simulink model "Model_pH_and_level_V1"  (Simulink 8.3)
settings: Solver=ode1  SolverMode=SingleTasking  StartTime=0.0  StopTime=Tsim  FixedStep=delta_sim  RelTol=1e-7
values from neighbouring files (symbols this model uses):
  b = 0    [Configuring_pH_and_level_model.m]
  delta_sim = 0.05    [Simulating_pH_and_level_model.m]
  e1 = 50    [Configuring_pH_and_level_model.m]
  e2 = 300    [Configuring_pH_and_level_model.m]
  filter_estimator1 = 1    [Configuring_pH_and_level_model.m]
  filter_estimator2 = 1    [Configuring_pH_and_level_model.m]
  filter_estimator3 = 1    [Configuring_pH_and_level_model.m]
  filter_estimator4 = 1    [Configuring_pH_and_level_model.m]
  filter_estimator5 = 1    [Configuring_pH_and_level_model.m]
  filter_estimator6 = 1    [Configuring_pH_and_level_model.m]
  filtro_Kp = fir1(5,1/50)    [Configuring_pH_and_level_model.m]
  filtro_med_F_TAPI = 1    [Configuring_pH_and_level_model.m]
  filtro_med_F_TASI = 1    [Configuring_pH_and_level_model.m]
  filtro_med_pH = 1    [Configuring_pH_and_level_model.m]
  filtro_Ti = fir1(5,1/50)    [Configuring_pH_and_level_model.m]
  h_max_TR_m = 0.5    [Configuring_pH_and_level_model.m]
  h_nom = 75    [Configuring_pH_and_level_model.m]
  I_l = 271.52    [Configuring_pH_and_level_model.m]
  K_meter_flow = 3600    [Configuring_pH_and_level_model.m]
  K_meter_level = 1    [Configuring_pH_and_level_model.m]
  K_meter_pH = 1    [Configuring_pH_and_level_model.m]
  Kc = 3.5    [Configuring_pH_and_level_model.m]
  Kn = 100/14    (= 7.14285714286)    [Configuring_pH_and_level_model.m]
  Kv = 11e-2    (= 0.11)    [Configuring_pH_and_level_model.m]
  mv0 = 50    [Configuring_pH_and_level_model.m]
  N = 1/500    (= 0.002)    [Configuring_pH_and_level_model.m]
  P_l = 11.65    [Configuring_pH_and_level_model.m]
  pH_nom = 7    [Configuring_pH_and_level_model.m]
  pka1_CH3COOH = interp1(Temp,pK_CH3COOH,T)    [Configuring_pH_and_level_model.m]
  pka1_H2CO3 = interp1(Temp,pK_H2CO3,T)    [Configuring_pH_and_level_model.m]
  pka1_H3PO4 = interp1(Temp,pK_H3PO4,T)    [Configuring_pH_and_level_model.m]
  pka1_NH4 = interp1(Temp,pK_NH4,T)    [Configuring_pH_and_level_model.m]
  pka2_H2CO3 = interp1(Temp,pK_HCO3,T)    [Configuring_pH_and_level_model.m]
  pka2_H3PO4 = interp1(Temp,pK_H2PO4,T)    [Configuring_pH_and_level_model.m]
  pka3_H3PO4 = interp1(Temp,pK_HPO4,T)    [Configuring_pH_and_level_model.m]
  pKw = interp1(Temp,pK_H2O,T)    [Configuring_pH_and_level_model.m]
  Q_ap_nom = 49/3600    (= 0.0136111111111)    [Configuring_pH_and_level_model.m]
  Qb_nom = c_HCl/c_NaOH*Q_ap_nom    (= 0.00412773748633)    [Configuring_pH_and_level_model.m]
  seed_noise_level = 12345    [Configuring_pH_and_level_model.m]
  seed_noise_pH = 67890    [Configuring_pH_and_level_model.m]
  seed_noise_Q_ap = 357    [Configuring_pH_and_level_model.m]
  seed_noise_Q_as = 349    [Configuring_pH_and_level_model.m]
  T_noise_level = 2    [Configuring_pH_and_level_model.m]
  T_noise_pH = 3    [Configuring_pH_and_level_model.m]
  T_PWM = 10    [Configuring_pH_and_level_model.m]
  tau_meter_flow = 1.4    [Configuring_pH_and_level_model.m]
  tau_meter_level = 16    [Configuring_pH_and_level_model.m]
  tau_meter_pH = 5    [Configuring_pH_and_level_model.m]
  Td = 120    [Configuring_pH_and_level_model.m]
  td_meter_flow = 3.5    [Configuring_pH_and_level_model.m]
  td_meter_level = 6    [Configuring_pH_and_level_model.m]
  td_meter_pH = 3.5    [Configuring_pH_and_level_model.m]
  Ti = 150    [Configuring_pH_and_level_model.m]
  Tmix = 1.34    [Configuring_pH_and_level_model.m]
  Ts = 0.5    [Simulating_pH_and_level_model.m]
  Ts_F_TAPI = 1    [Configuring_pH_and_level_model.m]
  Ts_F_TASI = 1    [Configuring_pH_and_level_model.m]
  Ts_Kp = 5    [Configuring_pH_and_level_model.m]
  Ts_pH_m = 1    [Configuring_pH_and_level_model.m]
  Ts_Ti = 5    [Configuring_pH_and_level_model.m]
  Ts_w1 = 1    [Configuring_pH_and_level_model.m]
  Ts_w2 = 1    [Configuring_pH_and_level_model.m]
  Ts_w3 = 1    [Configuring_pH_and_level_model.m]
  Ts_w4 = 1    [Configuring_pH_and_level_model.m]
  Ts_w5 = 1    [Configuring_pH_and_level_model.m]
  Ts_w6 = 25    [Configuring_pH_and_level_model.m]
  V0_CSTR = V_max_CSTR*h_nom/h_max_TR    (= 46.3491936722)    [Configuring_pH_and_level_model.m]
  V_max_CSTR = A_util_TR*h_max_TR_m*1000    (= 61.7989248962)    [Configuring_pH_and_level_model.m]
  var_noise_level = 1.1e-3    (= 0.0011)    [Configuring_pH_and_level_model.m]
  var_noise_pH = 6.25e-5    (= 6.25e-05)    [Configuring_pH_and_level_model.m]
  var_noise_Q_ap = 1.56e-2    (= 0.0156)    [Configuring_pH_and_level_model.m]
  var_noise_Q_as = 1.56e-2    (= 0.0156)    [Configuring_pH_and_level_model.m]
  Vm = 0.836    [Configuring_pH_and_level_model.m]
  w1_ff_tap = 0.0056    [Configuring_pH_and_level_model.m]
  w1_ff_tas = 0    [Configuring_pH_and_level_model.m]
  w1_ff_tbb = -0.0185    [Configuring_pH_and_level_model.m]
  w2_ff_tap = 0.5e-4    (= 5e-05)    [Configuring_pH_and_level_model.m]
  w2_ff_tbb = 0.5e-4    (= 5e-05)    [Configuring_pH_and_level_model.m]
  w3_ff_tap = 3e-4    (= 0.0003)    [Configuring_pH_and_level_model.m]
  w3_ff_tas = 3e-4    (= 0.0003)    [Configuring_pH_and_level_model.m]
  w3_ff_tbb = 3e-4    (= 0.0003)    [Configuring_pH_and_level_model.m]
  w4_ff_tap = 2e-4    (= 0.0002)    [Configuring_pH_and_level_model.m]
  w4_ff_tas = 2e-4    (= 0.0002)    [Configuring_pH_and_level_model.m]
  w4_ff_tbb = 2e-4    (= 0.0002)    [Configuring_pH_and_level_model.m]
  w_ap1 = c_HCl    (= 0.0055861204494)    [Configuring_pH_and_level_model.m]
  w_ap2 = c_CH3COOH_r    (= 0.0001)    [Configuring_pH_and_level_model.m]
  w_ap3 = c_H2CO3_r    (= 0.0009)    [Configuring_pH_and_level_model.m]
  w_ap4 = c_NH4    (= 0.0002)    [Configuring_pH_and_level_model.m]
  w_ap5 = c_H3PO4    (= 1e-05)    [Configuring_pH_and_level_model.m]
  w_as1 = 0    [Configuring_pH_and_level_model.m]
  w_as2 = c_CH3COOH    (= 0.00676612574825)    [Configuring_pH_and_level_model.m]
  w_as3 = c_H2CO3_r    (= 0.0009)    [Configuring_pH_and_level_model.m]
  w_as4 = c_NH4    (= 0.0002)    [Configuring_pH_and_level_model.m]
  w_as5 = c_H3PO4    (= 1e-05)    [Configuring_pH_and_level_model.m]
  w_b1 = -c_NaOH    (= -0.0184200924523)    [Configuring_pH_and_level_model.m]
  w_b2 = c_CH3COOH_r    (= 0.0001)    [Configuring_pH_and_level_model.m]
  w_b3 = c_H2CO3    (= 0.0005)    [Configuring_pH_and_level_model.m]
  w_b4 = c_NH4    (= 0.0002)    [Configuring_pH_and_level_model.m]
  w_b5 = c_H3PO4    (= 1e-05)    [Configuring_pH_and_level_model.m]
  w_fb_tap = [w1_ff_tap w2_ff_tap w3_ff_tap w4_ff_tap]    [Configuring_pH_and_level_model.m]
  w_fb_tas = [w1_ff_tas 0 w3_ff_tas w4_ff_tas]    [Configuring_pH_and_level_model.m]
  w_r1_0 = [w1_r1_0; c_CH3COOH_r; c_H2CO3_r; c_NH4; c_H3PO4]    [Configuring_pH_and_level_model.m]
  x_MV_pump = [0 10 20 40 50 60 80 100]    [Configuring_pH_and_level_model.m]
  y_Q_pump = Q_l_h/3600    [Configuring_pH_and_level_model.m]
libraries: simulink x6, simulink_extras x4
(part 2 of 2)

== system Model_pH_and_level_V1/pH controller/controller/FB/Calculo Parâmetros Cont. ==
  note: F(1+T(pH))
  w : Inport
  pH_sp : Inport  Port=2
  F_TAPI : Inport  Port=3
  F_TASI : Inport  Port=4
  Constant1 : Constant  Value=1/e1
  Constant2 : Constant  Value=1/e2
  Constant3 : Constant  Value=46.35
  Constant4 : Constant  Value=e1
  Constant5 : Constant  Value=e2
  Constant6 : Constant
  Constant7 : Constant  Value=46.35
  Constant8 : Constant
  Divide1 : Product  Inputs=*/
  Divide4 : Product  Inputs=*/
  Gain2 : Gain  Gain=1/3600
  Gain3 : Gain  Gain=1/3600
  Product1 : Product
  Product2 : Product  Inputs=3
  Product4 : Product
  Sum{1..2,4,12} (4 alike) : Sum
  Sum3 : Sum  Inputs=+-
  Sum6 : Sum  Inputs=-+
  T(pH_sp) : Subsystem
  1/Ti : Outport
  Kp : Outport  Port=2
  wires:
  Sum12/1 -> Product4/2
  F_TAPI/1 -> Gain2/1
  F_TASI/1 -> Gain3/1
  Constant6/1 -> Sum1/2
  T(pH_sp)/1(T(pH_sp)) -> Sum1/1
  Constant4/1 -> Product2/2, Sum4/1
  Constant5/1 -> Product2/3, Sum4/2
  Product2/1 -> Divide4/1
  Constant2/1 -> Sum2/2
  Sum4/1 -> Sum6/2
  Sum2/1 -> Product1/1
  Constant3/1 -> Product1/2
  Gain2/1 -> Sum12/1, T(pH_sp)/3(F_TAPI)
  Sum1/1 -> Product4/1
  Constant1/1 -> Sum2/1
  Constant7/1 -> Divide4/2
  Product4/1 -> Sum3/2, Product2/1
  Sum3/1 -> Kp/1
  Divide4/1 -> Sum6/1
  Product1/1 -> Sum3/1
  Gain3/1 -> Sum12/2, T(pH_sp)/4(F_TASI)
  pH_sp/1 -> T(pH_sp)/2(pH_sp)
  w/1 -> T(pH_sp)/1(w)
  Divide1/1 -> 1/Ti/1
  Sum6/1 -> Divide1/2
  Constant8/1 -> Divide1/1

== system Model_pH_and_level_V1/pH controller/controller/FB/T(pH) ==
  w : Inport
  pH : Inport  Port=2
  pH_sp : Inport  Port=3
  F_TAPI : Inport  Port=4
  F_TASI : Inport  Port=5
  Constant1 : Constant
  Constant5 : Constant
  Gain2 : Gain  Gain=1/3600
  Gain3 : Gain  Gain=1/3600
  Sum1 : Sum
  Sum2 : Sum
  Sum5 : Sum  Inputs=+-
  T(pH) : Subsystem
  T(pH_sp) : Subsystem
  1+T(pH_sp) : Outport
  T(pH_sp)-T(pH) : Outport  Port=2
  1+T(pH) : Outport  Port=3
  wires:
  w/1 -> T(pH)/1(w), T(pH_sp)/1(w)
  pH_sp/1 -> T(pH_sp)/2(pH_sp)
  Gain3/1 -> T(pH)/4(F_TASI), T(pH_sp)/4(F_TASI)
  Gain2/1 -> T(pH_sp)/3(F_TAPI), T(pH)/3(F_TAPI)
  F_TASI/1 -> Gain3/1
  F_TAPI/1 -> Gain2/1
  pH/1 -> T(pH)/2(pH)
  T(pH_sp)/1(T(pH_sp)) -> Sum1/2, Sum5/1
  T(pH)/1(T(pH)) -> Sum2/1, Sum5/2
  Constant5/1 -> Sum1/1
  Constant1/1 -> Sum2/2
  Sum5/1 -> T(pH_sp)-T(pH)/1
  Sum1/1 -> 1+T(pH_sp)/1
  Sum2/1 -> 1+T(pH)/1

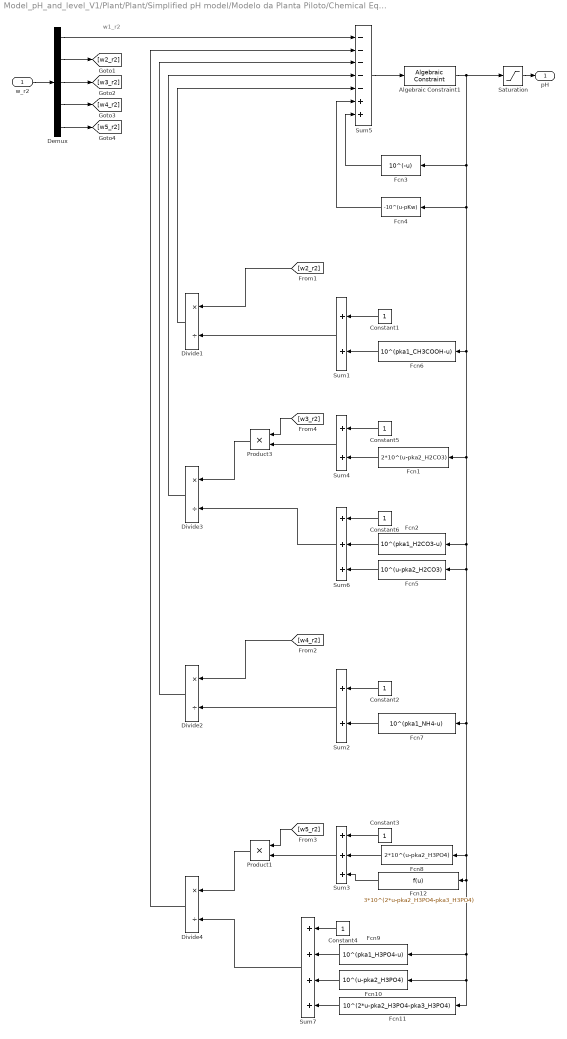
== system Model_pH_and_level_V1/Plant/Plant/Simplified pH model/Modelo da Planta Piloto/Chemical Equilibrium ==
  note: w1_r2
  w_r2 : Inport
  Algebraic Constraint1 : simulink/Math Operations/Algebraic Constraint  z0=7
  Constant{1..6} (6 alike) : Constant
  Demux : Demux  Outputs=5
  Divide{1..4} (4 alike) : Product  Inputs=*/
  Fcn1 : Fcn  Expr=2*10^(u-pka2_H2CO3)
  Fcn10 : Fcn  Expr=10^(u-pka2_H3PO4)
  Fcn11 : Fcn  Expr=10^(2*u-pka2_H3PO4-pka3_H3PO4)
  Fcn12 : Fcn  Expr=3*10^(2*u-pka2_H3PO4-pka3_H3PO4)
  Fcn2 : Fcn  Expr=10^(pka1_H2CO3-u)
  Fcn3 : Fcn  Expr=10^(-u)
  Fcn4 : Fcn  Expr=-10^(u-pKw)
  Fcn5 : Fcn  Expr=10^(u-pka2_H2CO3)
  Fcn6 : Fcn  Expr=10^(pka1_CH3COOH-u)
  Fcn7 : Fcn  Expr=10^(pka1_NH4-u)
  Fcn8 : Fcn  Expr=2*10^(u-pka2_H3PO4)
  Fcn9 : Fcn  Expr=10^(pka1_H3PO4-u)
  Product1 : Product
  Product3 : Product
  Saturation : Saturate  UpperLimit=14  LowerLimit=0
  Sum1 : Sum
  Sum2 : Sum
  Sum3 : Sum  Inputs=+++
  Sum4 : Sum
  Sum5 : Sum  Inputs=-----++
  Sum6 : Sum  Inputs=+++
  Sum7 : Sum  Inputs=++++
  pH : Outport
  wires:
  Sum4/1 -> Product3/2
  Product3/1 -> Divide3/1
  Constant5/1 -> Sum4/1
  Algebraic Constraint1/1 -> Fcn3/1, Fcn6/1, Fcn1/1, Fcn2/1, Fcn5/1, Fcn12/1, Fcn9/1, Fcn10/1, Fcn11/1, Fcn8/1, Fcn7/1, Fcn4/1, Saturation/1
  Fcn5/1 -> Sum6/3
  Sum6/1 -> Divide3/2
  Sum5/1 -> Algebraic Constraint1/1
  Fcn1/1 -> Sum4/2
  Fcn2/1 -> Sum6/2
  Constant6/1 -> Sum6/1
  Saturation/1 -> pH/1
  w_r2/1 -> Demux/1
  Demux/1 -> Sum5/1
  Demux/2 -> [w2_r2]
  Demux/3 -> [w3_r2]
  [w3_r2] -> Product3/1
  [w2_r2] -> Divide1/1
  Sum1/1 -> Divide1/2
  Fcn6/1 -> Sum1/2
  Constant1/1 -> Sum1/1
  Demux/4 -> [w4_r2]
  [w4_r2] -> Divide2/1
  Sum2/1 -> Divide2/2
  Fcn7/1 -> Sum2/2
  Constant2/1 -> Sum2/1
  Fcn3/1 -> Sum5/7
  Fcn4/1 -> Sum5/6
  Sum3/1 -> Product1/2
  Product1/1 -> Divide4/1
  Constant3/1 -> Sum3/1
  Fcn10/1 -> Sum7/3
  Sum7/1 -> Divide4/2
  Fcn8/1 -> Sum3/2
  Fcn9/1 -> Sum7/2
  Constant4/1 -> Sum7/1
  [w5_r2] -> Product1/1
  Fcn11/1 -> Sum7/4
  Demux/5 -> [w5_r2]
  Divide1/1 -> Sum5/5
  Divide3/1 -> Sum5/4
  Divide2/1 -> Sum5/3
  Divide4/1 -> Sum5/2
  Fcn12/1 -> Sum3/3

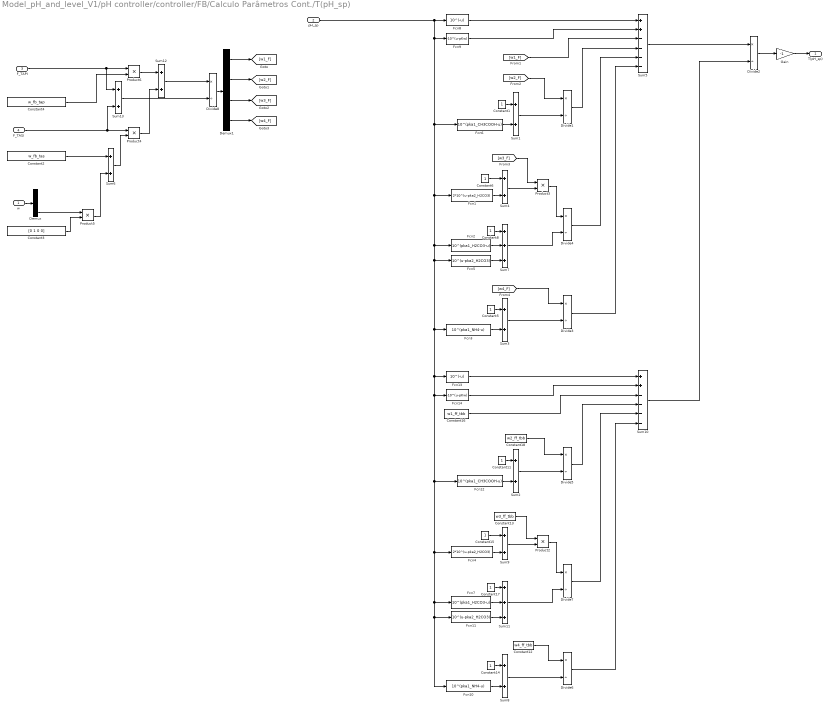
== system Model_pH_and_level_V1/pH controller/controller/FB/Calculo Parâmetros Cont./T(pH_sp) ==
  w : Inport
  pH_sp : Inport  Port=2
  F_TAPI : Inport  Port=3
  F_TASI : Inport  Port=4
  Constant{1,5..6,8,11,14..15,17} (8 alike) : Constant
  Constant12 : Constant  Value=w4_ff_tbb
  Constant13 : Constant  Value=w3_ff_tbb
  Constant16 : Constant  Value=w1_ff_tbb
  Constant18 : Constant  Value=w2_ff_tbb
  Constant2 : Constant  Value=w_fb_tas
  Constant3 : Constant  Value=[0 1 0 0]
  Constant4 : Constant  Value=w_fb_tap
  Demux : Demux  Outputs=6
  Demux1 : Demux
  Divide{1..8} (8 alike) : Product  Inputs=*/
  Fcn1 : Fcn  Expr=2*10^(u-pka2_H2CO3)
  Fcn10 : Fcn  Expr=10^(pka1_NH4-u)
  Fcn11 : Fcn  Expr=10^(u-pka2_H2CO3)
  Fcn12 : Fcn  Expr=10^(pka1_CH3COOH-u)
  Fcn13 : Fcn  Expr=10^(-u)
  Fcn14 : Fcn  Expr=-10^(u-pKw)
  Fcn2 : Fcn  Expr=10^(pka1_H2CO3-u)
  Fcn3 : Fcn  Expr=10^(pka1_NH4-u)
  Fcn4 : Fcn  Expr=2*10^(u-pka2_H2CO3)
  Fcn5 : Fcn  Expr=10^(u-pka2_H2CO3)
  Fcn6 : Fcn  Expr=10^(pka1_CH3COOH-u)
  Fcn7 : Fcn  Expr=10^(pka1_H2CO3-u)
  Fcn8 : Fcn  Expr=10^(-u)
  Fcn9 : Fcn  Expr=-10^(u-pKw)
  Gain : Gain  Gain=-1
  Product{2..4,6} (4 alike) : Product
  Product5 : Product  SampleTime=Ts_w5
  Sum{1..4,6,8..9,12..13} (9 alike) : Sum
  Sum10 : Sum  Inputs=++----
  Sum11 : Sum  Inputs=+++
  Sum5 : Sum  Inputs=++----
  Sum7 : Sum  Inputs=+++
  T(pH_sp) : Outport
  wires:
  Gain/1 -> T(pH_sp)/1
  w/1 -> Demux/1
  Constant18/1 -> Divide5/1
  Fcn7/1 -> Sum11/2
  Fcn4/1 -> Sum9/2
  Divide7/1 -> Sum10/5
  Sum10/1 -> Divide2/2
  Constant14/1 -> Sum8/1
  Constant12/1 -> Divide6/1
  Constant11/1 -> Sum2/1
  Fcn12/1 -> Sum2/2
  Sum2/1 -> Divide5/2
  Constant16/1 -> Sum10/3
  Divide6/1 -> Sum10/6
  Constant13/1 -> Product2/1
  Divide5/1 -> Sum10/4
  Constant17/1 -> Sum11/1
  Fcn13/1 -> Sum10/1
  Fcn10/1 -> Sum8/2
  Fcn14/1 -> Sum10/2
  Sum8/1 -> Divide6/2
  Fcn9/1 -> Sum5/2
  Fcn11/1 -> Sum11/3
  Sum11/1 -> Divide7/2
  Sum9/1 -> Product2/2
  pH_sp/1 -> Fcn8/1, Fcn9/1, Fcn6/1, Fcn1/1, Fcn2/1, Fcn3/1, Fcn10/1, Fcn11/1, Fcn7/1, Fcn4/1, Fcn12/1, Fcn14/1, Fcn13/1, Fcn5/1
  Divide4/1 -> Sum5/5
  Divide1/1 -> Sum5/4
  Sum5/1 -> Divide2/1
  Divide3/1 -> Sum5/6
  Constant15/1 -> Sum9/1
  [w4_F] -> Divide3/1
  Fcn3/1 -> Sum3/2
  [w2_F] -> Divide1/1
  Sum3/1 -> Divide3/2
  Product2/1 -> Divide7/1
  Fcn8/1 -> Sum5/1
  Constant5/1 -> Sum3/1
  Constant1/1 -> Sum1/1
  Sum4/1 -> Product3/2
  Fcn1/1 -> Sum4/2
  Fcn2/1 -> Sum7/2
  Sum1/1 -> Divide1/2
  Fcn6/1 -> Sum1/2
  Constant6/1 -> Sum4/1
  Sum7/1 -> Divide4/2
  Constant8/1 -> Sum7/1
  Fcn5/1 -> Sum7/3
  Product3/1 -> Divide4/1
  [w1_F] -> Sum5/3
  [w3_F] -> Product3/1
  F_TASI/1 -> Sum13/2, Product4/1
  Constant3/1 -> Product5/2
  Product5/1 -> Sum6/2
  Constant2/1 -> Sum6/1
  Sum6/1 -> Product4/2
  F_TAPI/1 -> Sum13/1, Product6/1
  Constant4/1 -> Product6/2
  Product6/1 -> Sum12/1
  Product4/1 -> Sum12/2
  Sum12/1 -> Divide8/1
  Sum13/1 -> Divide8/2
  Divide8/1 -> Demux1/1
  Demux1/1 -> [w1_F]
  Demux1/2 -> [w2_F]
  Demux1/3 -> [w3_F]
  Demux1/4 -> [w4_F]
  Divide2/1 -> Gain/1
  Demux/6 -> Product5/1

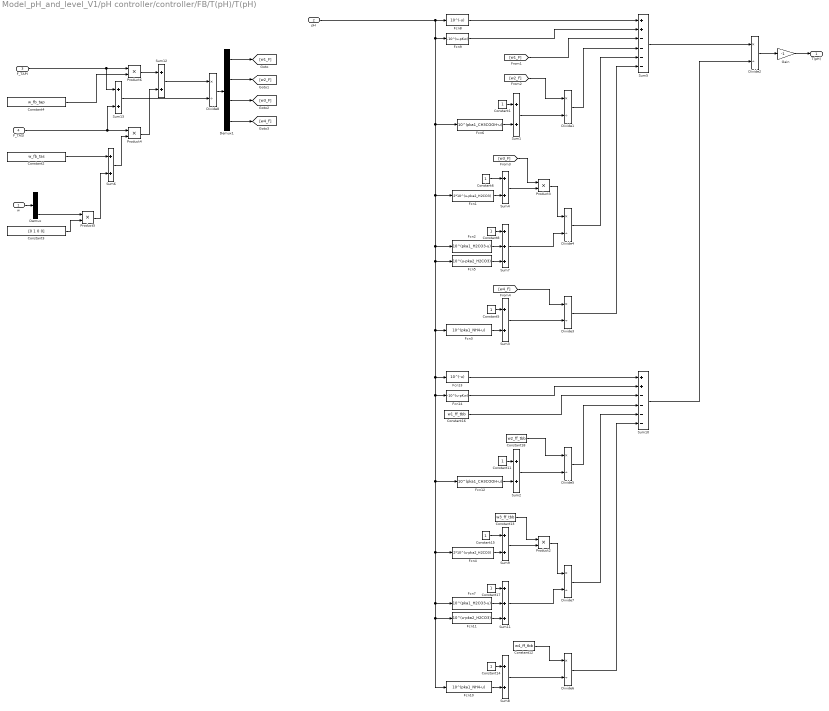
== system Model_pH_and_level_V1/pH controller/controller/FB/T(pH)/T(pH) ==
  w : Inport
  pH : Inport  Port=2
  F_TAPI : Inport  Port=3
  F_TASI : Inport  Port=4
  Constant{1,5..6,8,11,14..15,17} (8 alike) : Constant
  Constant12 : Constant  Value=w4_ff_tbb
  Constant13 : Constant  Value=w3_ff_tbb
  Constant16 : Constant  Value=w1_ff_tbb
  Constant18 : Constant  Value=w2_ff_tbb
  Constant2 : Constant  Value=w_fb_tas
  Constant3 : Constant  Value=[0 1 0 0]
  Constant4 : Constant  Value=w_fb_tap
  Demux : Demux  Outputs=6
  Demux1 : Demux
  Divide{1..8} (8 alike) : Product  Inputs=*/
  Fcn1 : Fcn  Expr=2*10^(u-pka2_H2CO3)
  Fcn10 : Fcn  Expr=10^(pka1_NH4-u)
  Fcn11 : Fcn  Expr=10^(u-pka2_H2CO3)
  Fcn12 : Fcn  Expr=10^(pka1_CH3COOH-u)
  Fcn13 : Fcn  Expr=10^(-u)
  Fcn14 : Fcn  Expr=-10^(u-pKw)
  Fcn2 : Fcn  Expr=10^(pka1_H2CO3-u)
  Fcn3 : Fcn  Expr=10^(pka1_NH4-u)
  Fcn4 : Fcn  Expr=2*10^(u-pka2_H2CO3)
  Fcn5 : Fcn  Expr=10^(u-pka2_H2CO3)
  Fcn6 : Fcn  Expr=10^(pka1_CH3COOH-u)
  Fcn7 : Fcn  Expr=10^(pka1_H2CO3-u)
  Fcn8 : Fcn  Expr=10^(-u)
  Fcn9 : Fcn  Expr=-10^(u-pKw)
  Gain : Gain  Gain=-1
  Product{2..6} (5 alike) : Product
  Sum{1..4,6,8..9,12..13} (9 alike) : Sum
  Sum10 : Sum  Inputs=++----
  Sum11 : Sum  Inputs=+++
  Sum5 : Sum  Inputs=++----
  Sum7 : Sum  Inputs=+++
  T(pH) : Outport
  wires:
  Gain/1 -> T(pH)/1
  w/1 -> Demux/1
  Constant18/1 -> Divide5/1
  Fcn7/1 -> Sum11/2
  Fcn4/1 -> Sum9/2
  Divide7/1 -> Sum10/5
  Sum10/1 -> Divide2/2
  Constant14/1 -> Sum8/1
  Constant12/1 -> Divide6/1
  Constant11/1 -> Sum2/1
  Fcn12/1 -> Sum2/2
  Sum2/1 -> Divide5/2
  Constant16/1 -> Sum10/3
  Divide6/1 -> Sum10/6
  Constant13/1 -> Product2/1
  Divide5/1 -> Sum10/4
  Constant17/1 -> Sum11/1
  Fcn13/1 -> Sum10/1
  Fcn10/1 -> Sum8/2
  Fcn14/1 -> Sum10/2
  Sum8/1 -> Divide6/2
  Fcn9/1 -> Sum5/2
  Fcn11/1 -> Sum11/3
  Sum11/1 -> Divide7/2
  Sum9/1 -> Product2/2
  pH/1 -> Fcn8/1, Fcn9/1, Fcn6/1, Fcn1/1, Fcn2/1, Fcn3/1, Fcn10/1, Fcn11/1, Fcn7/1, Fcn4/1, Fcn12/1, Fcn14/1, Fcn13/1, Fcn5/1
  Divide4/1 -> Sum5/5
  Divide1/1 -> Sum5/4
  Sum5/1 -> Divide2/1
  Divide3/1 -> Sum5/6
  Constant15/1 -> Sum9/1
  [w4_F] -> Divide3/1
  Fcn3/1 -> Sum3/2
  [w2_F] -> Divide1/1
  Sum3/1 -> Divide3/2
  Product2/1 -> Divide7/1
  Fcn8/1 -> Sum5/1
  Constant5/1 -> Sum3/1
  Constant1/1 -> Sum1/1
  Sum4/1 -> Product3/2
  Fcn1/1 -> Sum4/2
  Fcn2/1 -> Sum7/2
  Sum1/1 -> Divide1/2
  Fcn6/1 -> Sum1/2
  Constant6/1 -> Sum4/1
  Sum7/1 -> Divide4/2
  Constant8/1 -> Sum7/1
  Fcn5/1 -> Sum7/3
  Product3/1 -> Divide4/1
  [w1_F] -> Sum5/3
  [w3_F] -> Product3/1
  F_TASI/1 -> Sum13/2, Product4/1
  Constant3/1 -> Product5/2
  Product5/1 -> Sum6/2
  Constant2/1 -> Sum6/1
  Sum6/1 -> Product4/2
  F_TAPI/1 -> Sum13/1, Product6/1
  Constant4/1 -> Product6/2
  Product6/1 -> Sum12/1
  Product4/1 -> Sum12/2
  Sum12/1 -> Divide8/1
  Sum13/1 -> Divide8/2
  Divide8/1 -> Demux1/1
  Demux1/1 -> [w1_F]
  Demux1/2 -> [w2_F]
  Demux1/3 -> [w3_F]
  Demux1/4 -> [w4_F]
  Divide2/1 -> Gain/1
  Demux/6 -> Product5/1

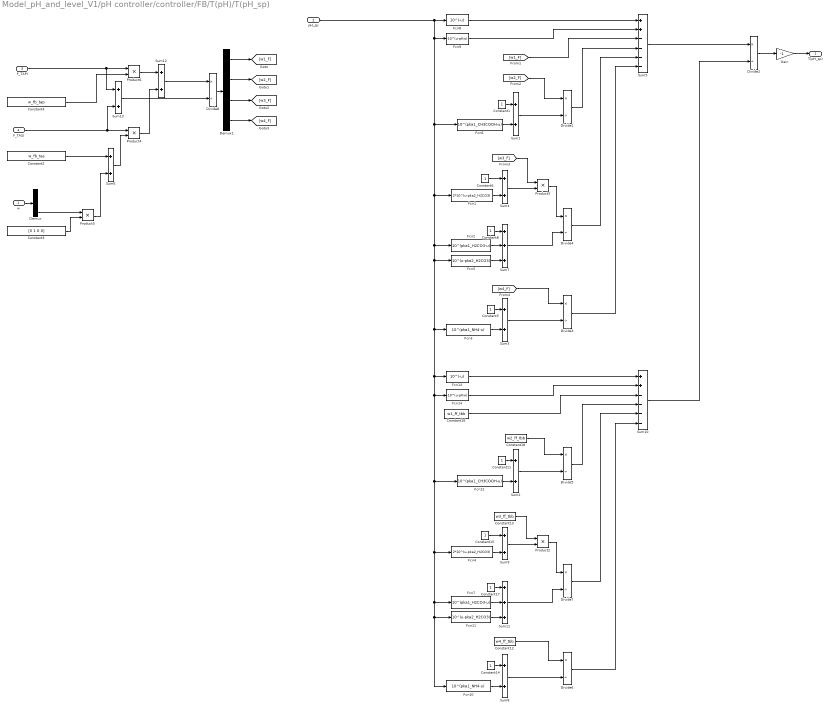
== system Model_pH_and_level_V1/pH controller/controller/FB/T(pH)/T(pH_sp) ==
  w : Inport
  pH_sp : Inport  Port=2
  F_TAPI : Inport  Port=3
  F_TASI : Inport  Port=4
  Constant{1,5..6,8,11,14..15,17} (8 alike) : Constant
  Constant12 : Constant  Value=w4_ff_tbb
  Constant13 : Constant  Value=w3_ff_tbb
  Constant16 : Constant  Value=w1_ff_tbb
  Constant18 : Constant  Value=w2_ff_tbb
  Constant2 : Constant  Value=w_fb_tas
  Constant3 : Constant  Value=[0 1 0 0]
  Constant4 : Constant  Value=w_fb_tap
  Demux : Demux  Outputs=6
  Demux1 : Demux
  Divide{1..8} (8 alike) : Product  Inputs=*/
  Fcn1 : Fcn  Expr=2*10^(u-pka2_H2CO3)
  Fcn10 : Fcn  Expr=10^(pka1_NH4-u)
  Fcn11 : Fcn  Expr=10^(u-pka2_H2CO3)
  Fcn12 : Fcn  Expr=10^(pka1_CH3COOH-u)
  Fcn13 : Fcn  Expr=10^(-u)
  Fcn14 : Fcn  Expr=-10^(u-pKw)
  Fcn2 : Fcn  Expr=10^(pka1_H2CO3-u)
  Fcn3 : Fcn  Expr=10^(pka1_NH4-u)
  Fcn4 : Fcn  Expr=2*10^(u-pka2_H2CO3)
  Fcn5 : Fcn  Expr=10^(u-pka2_H2CO3)
  Fcn6 : Fcn  Expr=10^(pka1_CH3COOH-u)
  Fcn7 : Fcn  Expr=10^(pka1_H2CO3-u)
  Fcn8 : Fcn  Expr=10^(-u)
  Fcn9 : Fcn  Expr=-10^(u-pKw)
  Gain : Gain  Gain=-1
  Product{2..6} (5 alike) : Product
  Sum{1..4,6,8..9,12..13} (9 alike) : Sum
  Sum10 : Sum  Inputs=++----
  Sum11 : Sum  Inputs=+++
  Sum5 : Sum  Inputs=++----
  Sum7 : Sum  Inputs=+++
  T(pH_sp) : Outport
  wires:
  Divide2/1 -> Gain/1
  Demux1/4 -> [w4_F]
  Demux1/3 -> [w3_F]
  Demux1/2 -> [w2_F]
  Demux1/1 -> [w1_F]
  Divide8/1 -> Demux1/1
  Sum13/1 -> Divide8/2
  Sum12/1 -> Divide8/1
  Product4/1 -> Sum12/2
  Product6/1 -> Sum12/1
  Constant4/1 -> Product6/2
  F_TAPI/1 -> Product6/1, Sum13/1
  Sum6/1 -> Product4/2
  Constant2/1 -> Sum6/1
  Product5/1 -> Sum6/2
  Constant3/1 -> Product5/2
  F_TASI/1 -> Product4/1, Sum13/2
  [w3_F] -> Product3/1
  [w1_F] -> Sum5/3
  Product3/1 -> Divide4/1
  Fcn5/1 -> Sum7/3
  Constant8/1 -> Sum7/1
  Sum7/1 -> Divide4/2
  Constant6/1 -> Sum4/1
  Fcn6/1 -> Sum1/2
  Sum1/1 -> Divide1/2
  Fcn2/1 -> Sum7/2
  Fcn1/1 -> Sum4/2
  Sum4/1 -> Product3/2
  Constant1/1 -> Sum1/1
  Constant5/1 -> Sum3/1
  Fcn8/1 -> Sum5/1
  Product2/1 -> Divide7/1
  Sum3/1 -> Divide3/2
  [w2_F] -> Divide1/1
  Fcn3/1 -> Sum3/2
  [w4_F] -> Divide3/1
  Constant15/1 -> Sum9/1
  Divide3/1 -> Sum5/6
  Sum5/1 -> Divide2/1
  Divide1/1 -> Sum5/4
  Divide4/1 -> Sum5/5
  pH_sp/1 -> Fcn5/1, Fcn13/1, Fcn14/1, Fcn12/1, Fcn4/1, Fcn7/1, Fcn11/1, Fcn10/1, Fcn3/1, Fcn2/1, Fcn1/1, Fcn6/1, Fcn9/1, Fcn8/1
  Sum9/1 -> Product2/2
  Sum11/1 -> Divide7/2
  Fcn11/1 -> Sum11/3
  Fcn9/1 -> Sum5/2
  Sum8/1 -> Divide6/2
  Fcn14/1 -> Sum10/2
  Fcn10/1 -> Sum8/2
  Fcn13/1 -> Sum10/1
  Constant17/1 -> Sum11/1
  Divide5/1 -> Sum10/4
  Constant13/1 -> Product2/1
  Divide6/1 -> Sum10/6
  Constant16/1 -> Sum10/3
  Sum2/1 -> Divide5/2
  Fcn12/1 -> Sum2/2
  Constant11/1 -> Sum2/1
  Constant12/1 -> Divide6/1
  Constant14/1 -> Sum8/1
  Sum10/1 -> Divide2/2
  Divide7/1 -> Sum10/5
  Fcn4/1 -> Sum9/2
  Fcn7/1 -> Sum11/2
  Constant18/1 -> Divide5/1
  w/1 -> Demux/1
  Gain/1 -> T(pH_sp)/1
  Demux/6 -> Product5/1
